simulink model "ContDiscintegral"  (R2023a)
settings: Solver=VariableStepAuto  StartTime=0.0  StopTime=5  RelTol=1e-3
undefined symbols (not defined in the file): DiscIntNeverNeededParam
settings Model: Creator=Egypt_Laptop  LastModifiedBy=Egypt_Laptop

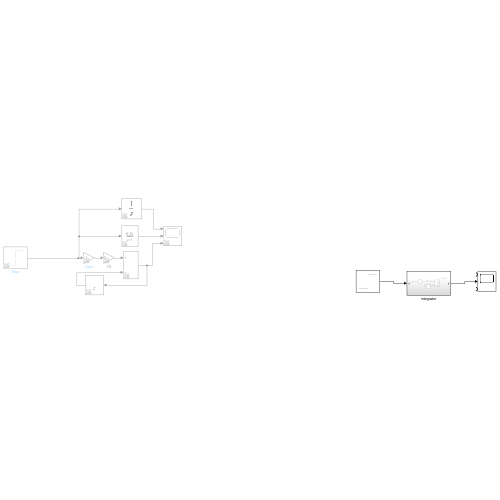
[thumbnail: Simulink's stored preview of the top-level diagram]
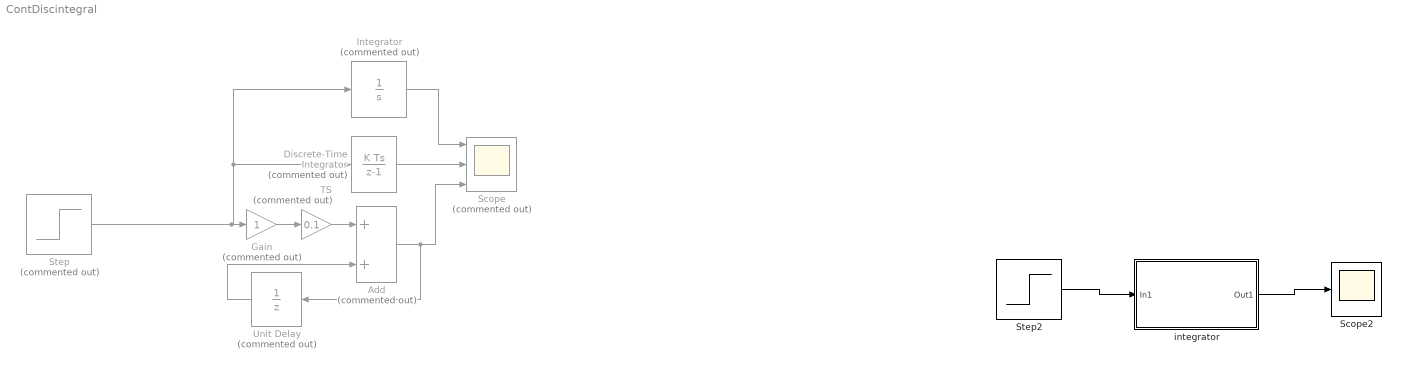
== system ContDiscintegral ==
  Add : Sum  Commented=on
  Discrete-Time Integrator : DiscreteIntegrator  Commented=on  SampleTime=-1  ICPrevOutput=DiscIntNeverNeededParam  ICPrevScaledInput=DiscIntNeverNeededParam
  Gain : Gain  Commented=on
  Integrator : Integrator  Commented=on
  Scope : Scope  Commented=on  NumInputPorts=3
  Scope2 : Scope  NumInputPorts=3
  Step : Step  Commented=on  SampleTime=0
  Step2 : Step  SampleTime=0
  TS : Gain  Commented=on  Gain=0.1
  Unit Delay : UnitDelay  Commented=on  SampleTime=-1  HasFrameUpgradeWarning=on
  integrator : Subsystem
  wires:
  Integrator/1 -> Scope/1
  TS/1 -> Add/1
  Unit Delay/1 -> Add/2
  Add/1 -> Unit Delay/1, Scope/3
  Discrete-Time Integrator/1 -> Scope/2
  Step/1 -> Gain/1, Integrator/1, Discrete-Time Integrator/1
  Gain/1 -> TS/1
  Step2/1 -> integrator/1(In1)
  integrator/1(Out1) -> Scope2/2

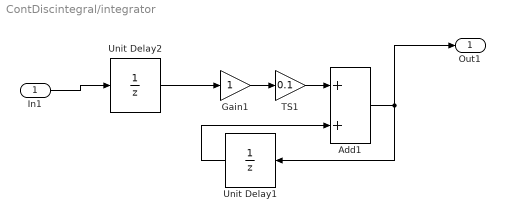
== system ContDiscintegral/integrator ==
  In1 : Inport
  Add1 : Sum
  Gain1 : Gain
  TS1 : Gain  Gain=0.1
  Unit Delay1 : UnitDelay  SampleTime=-1  HasFrameUpgradeWarning=on
  Unit Delay2 : UnitDelay  SampleTime=-1  HasFrameUpgradeWarning=on
  Out1 : Outport
  wires:
  Unit Delay2/1 -> Gain1/1
  Gain1/1 -> TS1/1
  TS1/1 -> Add1/1
  Add1/1 -> Out1/1, Unit Delay1/1
  In1/1 -> Unit Delay2/1
  Unit Delay1/1 -> Add1/2
